simulink model "gantry_crane_model"  (R2021b)
settings: Solver=FixedStepAuto  StartTime=0.0  StopTime=80  FixedStep=0.01  RelTol=1e-3
values from neighbouring files (symbols this model uses):
  f = 2    [gantry_crane_definitions.m]
  g = 9.81    [gantry_crane_definitions.m]
  l = 15    [gantry_crane_definitions.m]
  M = 50    [gantry_crane_definitions.m]
  m = 10    [gantry_crane_definitions.m]
  ts = tf/2    (= 35)    [gantry_crane_definitions.m]
undefined symbols (not defined in the file or in its folder): cf, hf, lf, M1, m1, magnitude
libraries: simulink x3
settings Model: Creator=AA  LastModifiedBy=AA

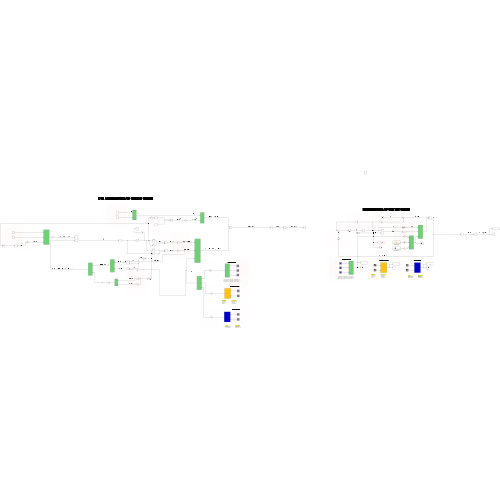
[thumbnail: Simulink's stored preview of the top-level diagram]
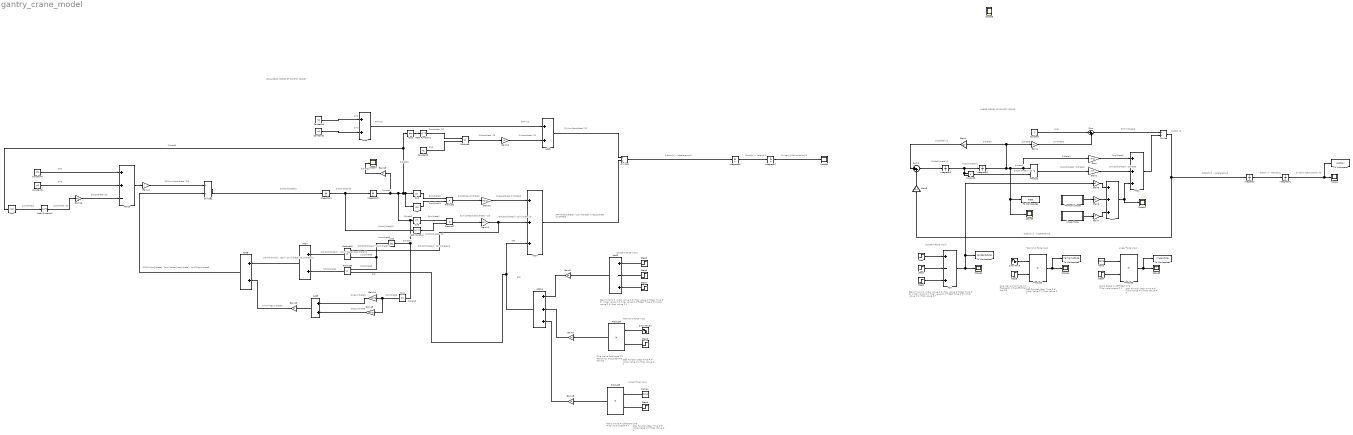
== system gantry_crane_model ==
  note: LINEAR MODEL OF GANTRY CRANE
  note: $mg\theta$
  note: $\ddot{x} - Acceleration$
  note: Step Time = 0, initial value = 0, final value = f
      | Step Time = ts, initial value = 0, final value = 2*f
      | Step Time = tf, initial value = 0, final value = f
  note: Constant Force Input
  note: $\dot{x} - Velocity$
  note: $x-\text {Cart position}$
  note: $ml\dot{\theta}^2\theta$
  note: $\theta$
  note: $\dot{\theta}^2\theta$
  note: $\theta$
  note: $\dot{\theta}^2$
  note: $\dot{\theta}$
  note: $\ddot{\theta}$
  note: $\theta$
  note: $m\theta$
  note: $M$
  note: $M+m\theta$
  note: $\ddot x$
  note: $\theta$
  note: $-g\theta /l$
  note: $\ddot{x} - Acceleration$
  note: Sine Wave
      | Amplitude = f
      | Frequency = $\pi/tf$
      | Phase = $\pi/2$
  note: Harmonic Force Input
  note: Step Function
      | Step Time = tf
      | Initial Value = 1
      | Final Value = 1
  note: Linear Force Input
  note: Step Function
      | Step Time = tf
      | Initial Value = 1
      | Final Value = 0
  note: Ramp
      | Slope = -2f/tf
      | Start time = 0s
      | Initial output = f
  note: $\dot{\theta}$
  note: $\ddot{\theta}$
  note: $\theta$
  note: $sin\theta$
  note: $cos\theta$
  note: $cos\theta sin\theta$
  note: $Mgcos\theta sin\theta$
  note: $\theta$
  note: $sin\theta$
  note: $\dot{\theta}^2$
  note: $\dot{\theta}$
  note: $sin{\theta}\dot{\theta}^2$
  note: $Ml\dot{\theta}^2sin{\theta}$
  note: $F+Ml\dot{\theta}^2sin{\theta}+ Mgcos\theta sin\theta$
  note: $M$
  note: $m$
  note: $M+m$
  note: $\theta$
  note: $cos\theta^2$
  note: $M$
  note: $M+m$
  note: $Mcos\theta^2$
  note: $-Mcos\theta^2$
  note: $M+m-Mcos\theta^2$
  note: $cos\theta$
  note: $F$
  note: $F$
  note: $cos\theta$
  note: $Ml\dot{\theta}^2sin{\theta}$
  note: $Ml\dot{\theta}^2sin{\theta}$
  note: $cos\theta$
  note: $Ml\dot{\theta}^2sin{\theta}cos{\theta}$
  note: $Fcos\theta$
  note: $(F+Ml\dot{\theta}^2sin{\theta})cos{\theta}$
  note: $\theta$
  note: $\theta$
  note: $sin\theta$
  note: $mgsin\theta$
  note: $Mgsin\theta$
  note: $-(m+M)gsin\theta$
  note: $(F+Ml\dot{\theta}^2sin{\theta})cos{\theta} -(m+M)gsin\theta$
  note: $M$
  note: $m$
  note: $\theta$
  note: $cos\theta$
  note: $cos\theta^2$
  note: $Mcos\theta^2$
  note: $l(M+m-Mcos\theta^2)$
  note: $x-\text {Cart position}$
  note: $\dot{x} - Velocity$
  note: $\ddot{x} - Acceleration$
  note: NON-LINEAR MODEL OF GANTRY CRANE
  note: $\theta$
  note: Step Time = 0, initial value = 0, final value = f
      | Step Time = ts, initial value = 0, final value = 2*f
      | Step Time = tf, initial value = 0, final value = f
  note: Constant Force Input
  note: Harmonic Force Input
  note: Sine Wave
      | Amplitude = f
      | Frequency = $\pi/tf$
      | Phase = $\pi/2$
  note: Step Function
      | Step Time = tf
      | Initial Value = 1
      | Final Value = 1
  note: Ramp
      | Slope = -2f/tf
      | Start time = 0s
      | Initial output = f
  note: Linear Force Input
  note: Step Function
      | Step Time = tf
      | Initial Value = 1
      | Final Value = 0
  note: $F$
  Add : Sum  Inputs=+-+
  Add{1..2,4,11} (4 alike) : Sum  Inputs=+++
  Add10 : Sum  Inputs=++-
  Add3 : Sum  Inputs=+-+
  Add{5..9} (5 alike) : Sum
  Constant : Constant  Value=M
  Constant1 : Constant  Value=M1
  Constant2 : Constant  Value=m1
  Constant3 : Constant  Value=M1
  Constant4 : Constant  Value=M1
  Constant5 : Constant  Value=m1
  Cos{1..4} (4 alike) : Trigonometry  Operator=cos
  Divide : Product  Inputs=/*
  Divide1 : Product  Inputs=/*
  Divide2 : Product  Inputs=/*
  Gain : Gain  Gain=m*g
  Gain1 : Gain  Gain=m*l
  Gain10 : Gain  Gain=M1*g
  Gain11 : Gain  Gain=M1*l
  Gain12 : Gain  Gain=-1
  Gain13 : Gain  Gain=-1
  Gain14 : Gain  Gain=m1*g
  Gain15 : Gain  Gain=M1*g
  Gain16 : Gain  Gain=M1
  Gain17 : Gain  Gain=l
  Gain18 : Gain  Gain=lf
  Gain19 : Gain  Gain=-1
  Gain2 : Gain  Gain=m
  Gain3 : Gain  Gain=-1/l
  Gain4 : Gain  Gain=-g/l
  Gain5 : Gain  Gain=cf
  Gain6 : Gain  Gain=hf
  Gain7 : Gain  Gain=lf
  Gain8 : Gain  Gain=cf
  Gain9 : Gain  Gain=hf
  Harmonic Force : Subsystem
  Integrator{,1..7} (8 alike) : Integrator
  Linear Force : Subsystem
  Math Function : Math  Operator=magnitude^2  SaturateOnIntegerOverflow=on
  Math Function1 : Math  Operator=magnitude^2  SaturateOnIntegerOverflow=on
  Math Function2 : Math  Operator=magnitude^2  SaturateOnIntegerOverflow=on
  Product{,1..10} (11 alike) : Product
  Ramp : simulink/Sources/Ramp  slope=-2*f/tf  start=0  InitialOutput=f
  Ramp1 : simulink/Sources/Ramp  slope=-2*f/tf  start=0  InitialOutput=f
  Scope{,1..8} (9 alike) : Scope
  Sin2 : Trigonometry
  Sin3 : Trigonometry
  Sin4 : Trigonometry
  Sine Wave : Sin  Amplitude=f  Frequency=pi/tf  Phase=pi/2  SampleTime=0
  Sine Wave1 : Sin  Amplitude=f  Frequency=pi/tf  Phase=pi/2  SampleTime=0
  Step : Step  Time=0  After=f  SampleTime=0
  Step1 : Step  Time=ts  After=2*f  SampleTime=0
  Step2 : Step  Time=tf  After=f  SampleTime=0
  Step{3..4,8..9} (4 alike) : Step  Time=tf  Before=1  After=0  SampleTime=0
  Step5 : Step  Time=0  After=f  SampleTime=0
  Step6 : Step  Time=ts  After=2*f  SampleTime=0
  Step7 : Step  Time=tf  After=f  SampleTime=0
  Sum : Sum  Inputs=|++
  Sum1 : Sum  Inputs=|++
  To Workspace : ToWorkspace  VariableName=position  SaveFormat=Timeseries  SampleTime=-1
  To Workspace1 : ToWorkspace  VariableName=constant_force  SaveFormat=Timeseries  SampleTime=-1
      settings: Save2DSignal=2-D array (concatenate along first dimension)
  To Workspace2 : ToWorkspace  VariableName=theta  SaveFormat=Timeseries  SampleTime=-1
      settings: Save2DSignal=2-D array (concatenate along first dimension)
  To Workspace3 : ToWorkspace  VariableName=harmonic_force  SaveFormat=Timeseries  SampleTime=-1
  To Workspace4 : ToWorkspace  VariableName=linear_force  SaveFormat=Timeseries  SampleTime=-1
  wires:
  Step/1 -> Add/1
  Step1/1 -> Add/2
  Step2/1 -> Add/3
  Integrator1/1 -> To Workspace/1, Scope/1
  Integrator/1 -> Integrator1/1
  Gain/1 -> Add1/1
  Gain1/1 -> Add1/2
  Product/1 -> Gain1/1
  Product1/1 -> Product/2
  Integrator2/1 -> Gain4/1, Gain2/1, Scope3/1, To Workspace2/1, Gain/1, Product/1
  Integrator3/1 -> Product1/2, Product1/1, Integrator2/1
  Sum1/1 -> Integrator3/1
  Gain2/1 -> Sum/2
  Constant/1 -> Sum/1
  Sum/1 -> Divide/1
  Add1/1 -> Divide/2
  Divide/1 -> Gain3/1, Integrator/1
  Gain4/1 -> Sum1/1
  Gain3/1 -> Sum1/2
  Step3/1 -> Product2/2
  Sine Wave/1 -> Product2/1
  Product2/1 -> To Workspace3/1, Scope4/1
  Product3/1 -> To Workspace4/1, Scope5/1
  Step4/1 -> Product3/2
  Ramp/1 -> Product3/1
  Gain5/1 -> Add2/1
  Harmonic Force/1(Out1) -> Gain6/1
  Gain6/1 -> Add2/2
  Linear Force/1(Out1) -> Gain7/1
  Gain7/1 -> Add2/3
  Add2/1 -> Add1/3, Scope2/1
  Integrator4/1 -> Math Function/1, Integrator5/1
  Sin2/1 -> Product6/1
  Cos1/1 -> Product6/2
  Product6/1 -> Gain10/1
  Gain10/1 -> Add4/1
  Product7/1 -> Gain11/1
  Sin3/1 -> Product7/1
  Divide2/1 -> Integrator4/1
  Math Function/1 -> Product7/2
  Add4/1 -> Divide1/2
  Constant1/1 -> Add5/1
  Constant2/1 -> Add5/2
  Add5/1 -> Add6/1
  Cos2/1 -> Math Function1/1
  Constant3/1 -> Product8/2
  Product8/1 -> Gain12/1
  Math Function1/1 -> Product8/1
  Gain12/1 -> Add6/2
  Add6/1 -> Divide1/1
  Cos3/1 -> Product9/1, Product10/2
  Add11/1 -> Product9/2, Add4/3
  Gain11/1 -> Product10/1, Add4/2
  Product10/1 -> Add7/1
  Product9/1 -> Add7/2
  Add7/1 -> Add8/1
  Gain13/1 -> Add8/2
  Sin4/1 -> Gain15/1, Gain14/1
  Gain15/1 -> Add9/2
  Gain14/1 -> Add9/1
  Add9/1 -> Gain13/1
  Add8/1 -> Divide2/2
  Constant4/1 -> Add10/1
  Constant5/1 -> Add10/2
  Cos4/1 -> Math Function2/1
  Math Function2/1 -> Gain16/1
  Gain16/1 -> Add10/3
  Add10/1 -> Gain17/1
  Gain17/1 -> Divide2/1
  Divide1/1 -> Integrator6/1
  Integrator6/1 -> Integrator7/1
  Integrator7/1 -> Scope6/1
  Integrator5/1 -> Gain19/1, Cos2/1, Cos4/1, Cos1/1, Sin2/1, Sin3/1, Sin4/1, Cos3/1
  Step5/1 -> Add3/1
  Step6/1 -> Add3/2
  Step7/1 -> Add3/3
  Step8/1 -> Product4/2
  Sine Wave1/1 -> Product4/1
  Product4/1 -> Gain9/1
  Add3/1 -> Gain8/1
  Step9/1 -> Product5/2
  Ramp1/1 -> Product5/1
  Product5/1 -> Gain18/1
  Gain8/1 -> Add11/1
  Gain9/1 -> Add11/2
  Gain18/1 -> Add11/3
  Gain19/1 -> Scope7/1
  Add/1 -> Scope1/1, Gain5/1, To Workspace1/1

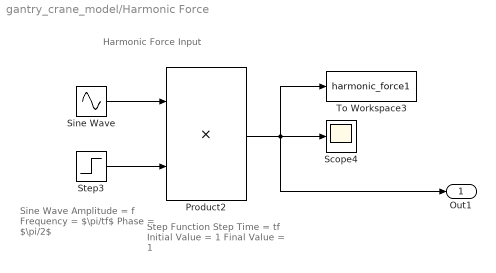
== system gantry_crane_model/Harmonic Force ==
  note: Harmonic Force Input
  note: Step Function
      | Step Time = tf
      | Initial Value = 1
      | Final Value = 1
  note: Sine Wave
      | Amplitude = f
      | Frequency = $\pi/tf$
      | Phase = $\pi/2$
  Product2 : Product
  Scope4 : Scope
  Sine Wave : Sin  Amplitude=f  Frequency=pi/tf  Phase=pi/2  SampleTime=0
  Step3 : Step  Time=tf  Before=1  After=0  SampleTime=0
  To Workspace3 : ToWorkspace  VariableName=harmonic_force1  SaveFormat=Timeseries  SampleTime=-1
  Out1 : Outport
  wires:
  Product2/1 -> Out1/1, To Workspace3/1, Scope4/1
  Step3/1 -> Product2/2
  Sine Wave/1 -> Product2/1

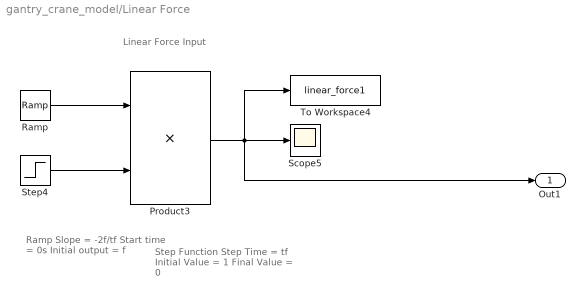
== system gantry_crane_model/Linear Force ==
  note: Ramp
      | Slope = -2f/tf
      | Start time = 0s
      | Initial output = f
  note: Step Function
      | Step Time = tf
      | Initial Value = 1
      | Final Value = 0
  note: Linear Force Input
  Product3 : Product
  Ramp : simulink/Sources/Ramp  slope=-2*f/tf  start=0  InitialOutput=f
  Scope5 : Scope
  Step4 : Step  Time=tf  Before=1  After=0  SampleTime=0
  To Workspace4 : ToWorkspace  VariableName=linear_force1  SaveFormat=Timeseries  SampleTime=-1
  Out1 : Outport
  wires:
  Product3/1 -> Out1/1, To Workspace4/1, Scope5/1
  Ramp/1 -> Product3/1
  Step4/1 -> Product3/2
